simulink model "METI_TM_CNT"  (R2018b)
settings: Solver=ode8  StartTime=0  StopTime=end_time  FixedStep=0.01  RelTol=1e-3
PreLoadFcn:
  | METI_TM_CNT_PreLoad;
undefined symbols (not defined in the file or in its folder): K2degC, TM_CNT_CVT_radpmin_min_rpm, TM_CNT_CVT_ratio_LL, TM_CNT_CVT_ratio_UL, TM_CNT_CVTFwarmer2_KpW, TM_CNT_CVTFwarmer2_KpW_x_T_CVTF, TM_CNT_CVTFwarmer_cold_Coolant_KpW, TM_CNT_CVTFwarmer_KpW, TM_CNT_CVTFwarmer_KpW_x_T_ENGCoolant, TM_CNT_CVTpritgt_rpm_table, TM_CNT_CVTpritgt_rpm_table_x_TVO, TM_CNT_delta_CVT_ratio_LL, TM_CNT_delta_CVT_ratio_UL, TM_CNT_Gain_CVT_ECU, TM_CNT_LU_Clutch_RelayOFF_rpm, TM_CNT_LU_Clutch_RelayON_rpm, TM_CNT_LU_slip_rpm_map, TM_CNT_LU_slip_rpm_map_x_speed_kmph, TM_CNT_LU_slip_rpm_map_y_TVO
libraries: simulink x2
settings Model: Creator=nishimura  LastModifiedBy=E00026
settings DataIOCC: LimitDataPoints=on  SaveFormat=Array  SaveOutput=off  InspectSignalLogs=on  SaveTime=off
settings OptimizationCC: BlockReduction=off  BooleanDataType=off  LifeSpan=inf
settings DebuggingCC: SaveWithParameterizedLinksMsg=none  UnderspecifiedInitializationDetection=Classic  MergeDetectMultiDrivingBlocksExec=none  SignalResolutionControl=TryResolveAllWithWarning  StrictBusMsg=ErrorOnBusTreatedAsVector  SFUnexpectedBacktrackingDiag=warning  SFNoUnconditionalDefaultTransitionDiag=warning  SFExecutionAtInitializationDiag=none
settings HardwareCC: ProdBitPerPointer=32  ProdBitPerSizeT=32  ProdBitPerPtrDiffT=32  ProdLargestAtomicFloat=None  ProdIntDivRoundTo=Undefined  ProdEndianess=Unspecified  ProdWordSize=32  ProdHWDeviceType=32-bit Generic  TargetUnknown=on
settings ModelReferenceCC: PropagateSignalLabelsOutOfModel=off
settings SFSimCC: SimUseLocalCustomCode=off
settings RTWCC: RTWUseLocalCustomCode=off
settings CodeAppCC: StateflowObjectComments=on
settings GRTTargetCC: TargetLangStandard=C89/C90 (ANSI)  GeneratePreprocessorConditionals=Disable all
settings ConfigComp: CovMetricSettings=dw  CovHtmlReporting=on  CovSaveCumulativeToWorkspaceVar=on  CovSaveSingleToWorkspaceVar=on  CovExternalEMLEnable=off  CovSFcnEnable=off

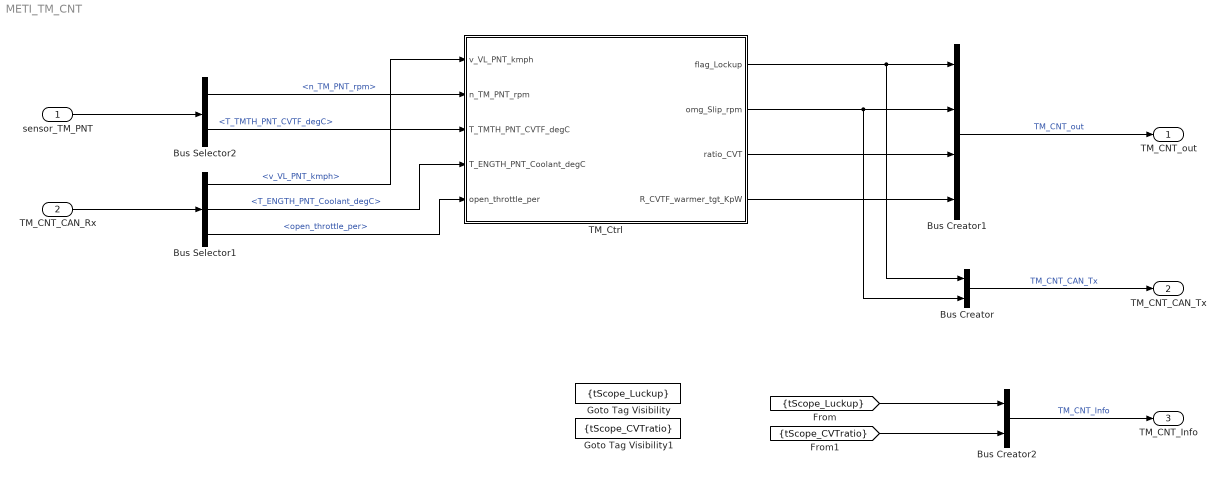
== system METI_TM_CNT ==
  sensor_TM_PNT : Inport  OutDataTypeStr=Bus: sensor_TM_PNT  SampleTime=0.01
      settings: AttributesFormatString=|
      | <SampleTime = %<SampleTime>>
      | <%<OutDataTypeStr>>
  TM_CNT_CAN_Rx : Inport  Port=2  OutDataTypeStr=Bus: TM_CNT_CAN_Rx  SampleTime=0.01
      settings: AttributesFormatString=|
      | <SampleTime = %<SampleTime>>
      | <%<OutDataTypeStr>>
  Bus Creator : BusCreator  Inputs=2
  Bus Creator1 : BusCreator  Inputs=4
  Bus Creator2 : BusCreator  Inputs=2
  Bus Selector1 : BusSelector  OutputSignals=v_VL_PNT_kmph,T_ENGTH_PNT_Coolant_degC,open_throttle_per
  Bus Selector2 : BusSelector  OutputSignals=n_TM_PNT_rpm,T_TMTH_PNT_CVTF_degC
  Goto Tag Visibility : GotoTagVisibility  GotoTag=tScope_Luckup
  Goto Tag Visibility1 : GotoTagVisibility  GotoTag=tScope_CVTratio
  TM_Ctrl : Subsystem
  TM_CNT_out : Outport  OutDataTypeStr=Bus: TM_CNT_out
      settings: AttributesFormatString=|
      | <SampleTime = %<SampleTime>>
      | <%<OutDataTypeStr>>
  TM_CNT_CAN_Tx : Outport  Port=2  OutDataTypeStr=Bus: TM_CNT_CAN_Tx
      settings: AttributesFormatString=|
      | <SampleTime = %<SampleTime>>
      | <%<OutDataTypeStr>>
  TM_CNT_Info : Outport  Port=3  OutDataTypeStr=Bus: TM_CNT_Info
      settings: AttributesFormatString=|
      | <SampleTime = %<SampleTime>>
      | <%<OutDataTypeStr>>
  wires:
  Bus Selector2/2 -> TM_Ctrl/3(T_TMTH_PNT_CVTF_degC)  "<T_TMTH_PNT_CVTF_degC>"
  Bus Selector1/3 -> TM_Ctrl/5(open_throttle_per)  "<open_throttle_per>"
  TM_Ctrl/2(omg_Slip_rpm) -> Bus Creator/2, Bus Creator1/2
  Bus Selector1/1 -> TM_Ctrl/1(v_VL_PNT_kmph)  "<v_VL_PNT_kmph>"
  [tScope_Luckup] -> Bus Creator2/1
  TM_Ctrl/1(flag_Lockup) -> Bus Creator/1, Bus Creator1/1
  [tScope_CVTratio] -> Bus Creator2/2
  Bus Selector2/1 -> TM_Ctrl/2(n_TM_PNT_rpm)  "<n_TM_PNT_rpm>"
  TM_Ctrl/3(ratio_CVT) -> Bus Creator1/3
  Bus Creator1/1 -> TM_CNT_out/1  "TM_CNT_out"
  sensor_TM_PNT/1 -> Bus Selector2/1
  TM_Ctrl/4(R_CVTF_warmer_tgt_KpW) -> Bus Creator1/4
  Bus Selector1/2 -> TM_Ctrl/4(T_ENGTH_PNT_Coolant_degC)  "<T_ENGTH_PNT_Coolant_degC>"
  Bus Creator2/1 -> TM_CNT_Info/1  "TM_CNT_Info"
  TM_CNT_CAN_Rx/1 -> Bus Selector1/1
  Bus Creator/1 -> TM_CNT_CAN_Tx/1  "TM_CNT_CAN_Tx"

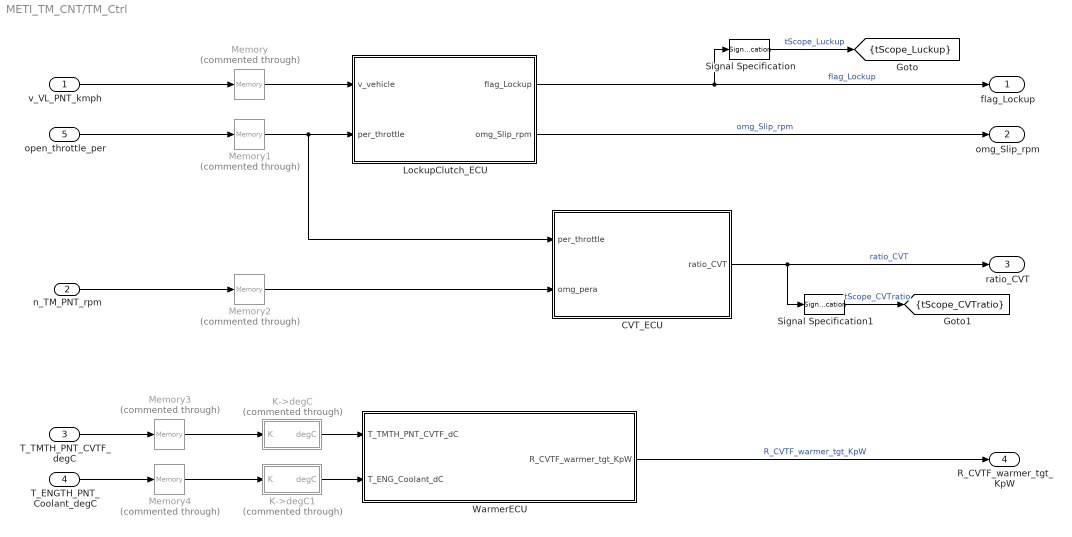
== system METI_TM_CNT/TM_Ctrl ==
  v_VL_PNT_kmph : Inport
  n_TM_PNT_rpm : Inport  Port=2
  T_TMTH_PNT_CVTF_degC : Inport  Port=3
  T_ENGTH_PNT_Coolant_degC : Inport  Port=4
  open_throttle_per : Inport  Port=5
  CVT_ECU : Subsystem
  K->degC : Subsystem  Commented=through
  K->degC1 : Subsystem  Commented=through
  LockupClutch_ECU : Subsystem
  Memory{,1..4} (5 alike) : Memory  Commented=through
  Signal Specification : SignalSpecification
  Signal Specification1 : SignalSpecification
  WarmerECU : Subsystem
  flag_Lockup : Outport
  omg_Slip_rpm : Outport  Port=2
  ratio_CVT : Outport  Port=3
  R_CVTF_warmer_tgt_KpW : Outport  Port=4
  tag scope: tScope_CVTratio=scoped, tScope_Luckup=scoped
  wires:
  Signal Specification1/1 -> [tScope_CVTratio]  "tScope_CVTratio"
  Signal Specification/1 -> [tScope_Luckup]  "tScope_Luckup"
  K->degC1/1(degC) -> WarmerECU/2(T_ENG_Coolant_dC)
  K->degC/1(degC) -> WarmerECU/1(T_TMTH_PNT_CVTF_dC)
  WarmerECU/1(R_CVTF_warmer_tgt_KpW) -> R_CVTF_warmer_tgt_KpW/1  "R_CVTF_warmer_tgt_KpW"
  Memory4/1 -> K->degC1/1(K)
  Memory3/1 -> K->degC/1(K)
  T_ENGTH_PNT_Coolant_degC/1 -> Memory4/1
  T_TMTH_PNT_CVTF_degC/1 -> Memory3/1
  v_VL_PNT_kmph/1 -> Memory/1
  n_TM_PNT_rpm/1 -> Memory2/1
  Memory2/1 -> CVT_ECU/2(omg_pera)
  Memory1/1 -> LockupClutch_ECU/2(per_throttle), CVT_ECU/1(per_throttle)
  Memory/1 -> LockupClutch_ECU/1(v_vehicle)
  open_throttle_per/1 -> Memory1/1
  LockupClutch_ECU/2(omg_Slip_rpm) -> omg_Slip_rpm/1  "omg_Slip_rpm"
  LockupClutch_ECU/1(flag_Lockup) -> flag_Lockup/1, Signal Specification/1  "flag_Lockup"
  CVT_ECU/1(ratio_CVT) -> ratio_CVT/1, Signal Specification1/1  "ratio_CVT"

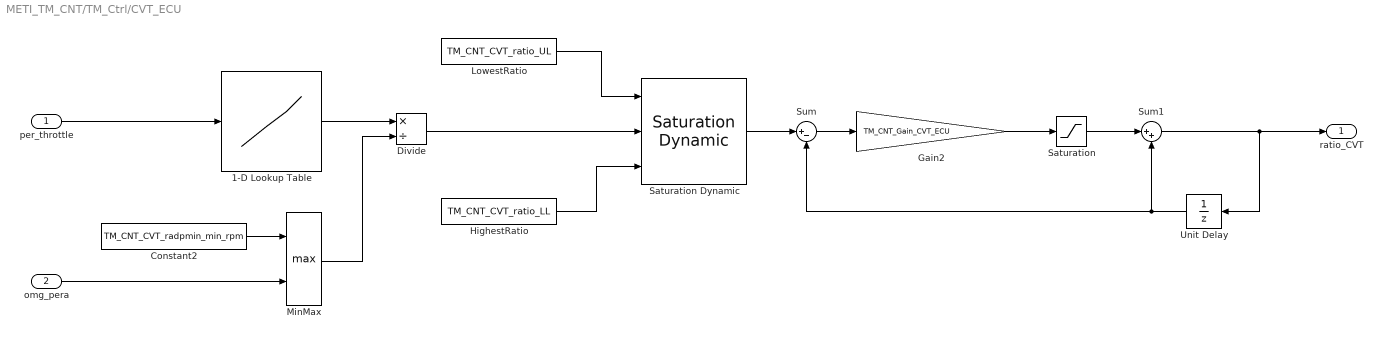
== system METI_TM_CNT/TM_Ctrl/CVT_ECU ==
  per_throttle : Inport
  omg_pera : Inport  Port=2
  1-D Lookup Table : Lookup_n-D  NumberOfTableDimensions=1  BreakpointsForDimension1=TM_CNT_CVTpritgt_rpm_table_x_TVO  Table=TM_CNT_CVTpritgt_rpm_table  RndMeth=Simplest  InputSameDT=on
  Constant2 : Constant  Value=TM_CNT_CVT_radpmin_min_rpm
  Divide : Product  Inputs=*/
  Gain2 : Gain  Gain=TM_CNT_Gain_CVT_ECU
  HighestRatio : Constant  Value=TM_CNT_CVT_ratio_LL
  LowestRatio : Constant  Value=TM_CNT_CVT_ratio_UL
  MinMax : MinMax  Function=max  Inputs=2
  Saturation : Saturate  UpperLimit=TM_CNT_delta_CVT_ratio_UL  LowerLimit=TM_CNT_delta_CVT_ratio_LL
  Saturation Dynamic : simulink/Discontinuities/Saturation Dynamic  OutMin=[]  OutMax=[]  OutDataTypeStr=Inherit: Same as second input  OutDataType=fixdt(1, 16)  OutScaling=2^-10  DoSatur=off
  Sum : Sum  Inputs=|+-
  Sum1 : Sum  Inputs=|++
  Unit Delay : UnitDelay  InitialCondition=1  SampleTime=-1
  ratio_CVT : Outport
  wires:
  Constant2/1 -> MinMax/1
  Saturation/1 -> Sum1/1
  omg_pera/1 -> MinMax/2
  per_throttle/1 -> 1-D Lookup Table/1
  Gain2/1 -> Saturation/1
  Sum/1 -> Gain2/1
  Sum1/1 -> Unit Delay/1, ratio_CVT/1
  Unit Delay/1 -> Sum/2, Sum1/2
  Saturation Dynamic/1 -> Sum/1
  MinMax/1 -> Divide/2
  HighestRatio/1 -> Saturation Dynamic/3
  LowestRatio/1 -> Saturation Dynamic/1
  Divide/1 -> Saturation Dynamic/2
  1-D Lookup Table/1 -> Divide/1

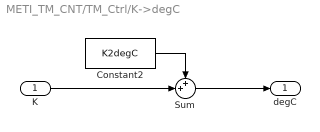
== system METI_TM_CNT/TM_Ctrl/K->degC ==
  K : Inport
  Constant2 : Constant  Value=K2degC
  Sum : Sum  Inputs=++|
  degC : Outport
  wires:
  K/1 -> Sum/2
  Constant2/1 -> Sum/1
  Sum/1 -> degC/1

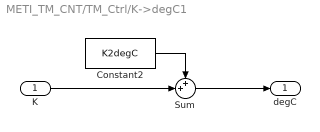
== system METI_TM_CNT/TM_Ctrl/K->degC1 ==
  K : Inport
  Constant2 : Constant  Value=K2degC
  Sum : Sum  Inputs=++|
  degC : Outport
  wires:
  Sum/1 -> degC/1
  Constant2/1 -> Sum/1
  K/1 -> Sum/2

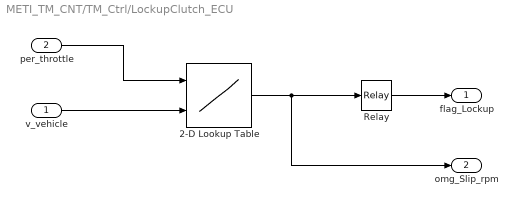
== system METI_TM_CNT/TM_Ctrl/LockupClutch_ECU ==
  v_vehicle : Inport
  per_throttle : Inport  Port=2
  2-D Lookup Table : Lookup_n-D  BreakpointsForDimension1=TM_CNT_LU_slip_rpm_map_y_TVO  BreakpointsForDimension2=TM_CNT_LU_slip_rpm_map_x_speed_kmph  Table=TM_CNT_LU_slip_rpm_map  RndMeth=Simplest  InputSameDT=on
  Relay : Relay  OnSwitchValue=TM_CNT_LU_Clutch_RelayON_rpm  OffSwitchValue=TM_CNT_LU_Clutch_RelayOFF_rpm  OnOutputValue=0  OffOutputValue=1
  flag_Lockup : Outport
  omg_Slip_rpm : Outport  Port=2
  wires:
  Relay/1 -> flag_Lockup/1
  per_throttle/1 -> 2-D Lookup Table/1
  2-D Lookup Table/1 -> Relay/1, omg_Slip_rpm/1
  v_vehicle/1 -> 2-D Lookup Table/2

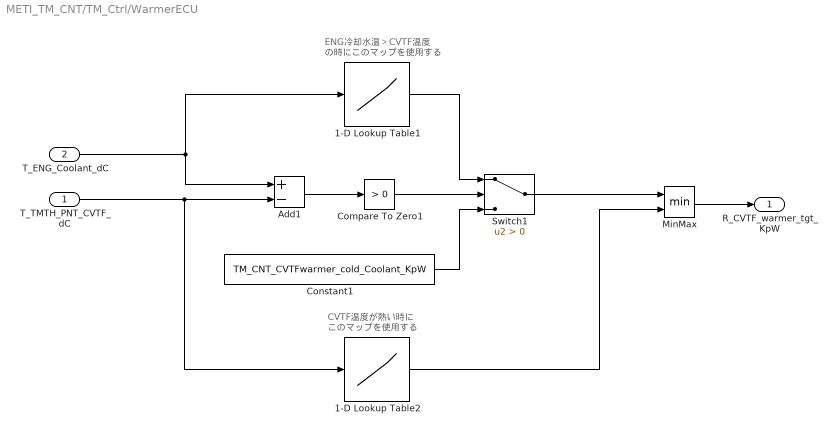
== system METI_TM_CNT/TM_Ctrl/WarmerECU ==
  note: CVTF温度が熱い時に
      | このマップを使用する
  note: ENG冷却水温＞CVTF温度
      | の時にこのマップを使用する
  T_TMTH_PNT_CVTF_dC : Inport
  T_ENG_Coolant_dC : Inport  Port=2
  1-D Lookup Table1 : Lookup_n-D  NumberOfTableDimensions=1  BreakpointsForDimension1=TM_CNT_CVTFwarmer_KpW_x_T_ENGCoolant  BeginIndexSearchUsingPreviousIndexResult=on  Table=TM_CNT_CVTFwarmer_KpW  ExtrapMethod=Clip  InternalRulePriority=Speed  RndMeth=Simplest  InputSameDT=on
  1-D Lookup Table2 : Lookup_n-D  NumberOfTableDimensions=1  BreakpointsForDimension1=TM_CNT_CVTFwarmer2_KpW_x_T_CVTF  BeginIndexSearchUsingPreviousIndexResult=on  Table=TM_CNT_CVTFwarmer2_KpW  ExtrapMethod=Clip  InternalRulePriority=Speed  RndMeth=Simplest  InputSameDT=on
  Add1 : Sum  Inputs=+-
  Compare To Zero1 : simulink/Logic and Bit Operations/Compare To Zero  relop=>  OutDataTypeStr=boolean
  Constant1 : Constant  Value=TM_CNT_CVTFwarmer_cold_Coolant_KpW
  MinMax : MinMax  Inputs=2
  Switch1 : Switch  Criteria=u2 > Threshold
  R_CVTF_warmer_tgt_KpW : Outport
  wires:
  1-D Lookup Table2/1 -> MinMax/2
  Switch1/1 -> MinMax/1
  T_TMTH_PNT_CVTF_dC/1 -> Add1/2, 1-D Lookup Table2/1
  T_ENG_Coolant_dC/1 -> Add1/1, 1-D Lookup Table1/1
  Constant1/1 -> Switch1/3
  1-D Lookup Table1/1 -> Switch1/1
  Compare To Zero1/1 -> Switch1/2
  Add1/1 -> Compare To Zero1/1
  MinMax/1 -> R_CVTF_warmer_tgt_KpW/1
